simulink model "sl_sfun"  (R2015b)
settings: Solver=VariableStepAuto  StartTime=0.0  StopTime=10.0  RelTol=1e-3
settings Model: Creator=zihan  LastModifiedBy=zihan

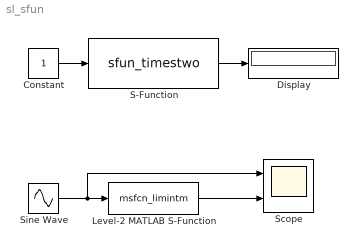
== system sl_sfun ==
  Constant : Constant
  Display : Display
  Level-2 MATLAB S-Function : M-S-Function  FunctionName=msfcn_limintm  Parameters=-5 5 0
  S-Function : S-Function  FunctionName=sfun_timestwo  SFunctionDeploymentMode=off  EnableBusSupport=off
  Scope : Scope  NumInputPorts=2
  Sine Wave : Sin  Amplitude=10  SampleTime=0
  wires:
  Constant/1 -> S-Function/1
  S-Function/1 -> Display/1
  Sine Wave/1 -> Scope/1, Level-2 MATLAB S-Function/1
  Level-2 MATLAB S-Function/1 -> Scope/2
